simulink model "elevator"  (R2020a)
settings: Solver=FixedStepAuto  StartTime=0.0  StopTime=100  FixedStep=0.001  RelTol=1e-3
settings Model: EnablePacing=on  Creator=Main  LastModifiedBy=Main
settings SolverCC: ZeroCrossAlgorithm=Adaptive
settings DebuggingCC: IgnoredZcDiagnostic=none
settings RTWCC: GenCodeOnly=on  PackageGeneratedCodeAndArtifacts=on
settings GRTTargetCC: MatFileLogging=off
settings ConfigComp: DVTestSuiteOptimization=Auto  DVDetectOutOfBounds=on

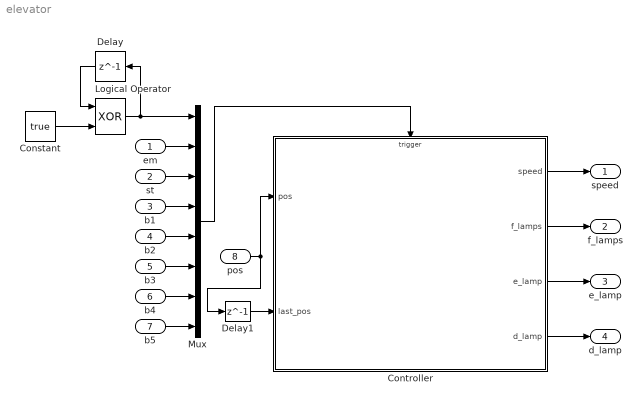
== system elevator ==
  em : Inport
  st : Inport  Port=2
  b1 : Inport  Port=3
  b2 : Inport  Port=4
  b3 : Inport  Port=5
  b4 : Inport  Port=6
  b5 : Inport  Port=7
  pos : Inport  Port=8
  Constant : Constant  Value=true  OutDataTypeStr=boolean
  Controller : Stateflow chart  TreatAsAtomicUnit=on
  Delay : Delay  DelayLength=1
  Delay1 : Delay  DelayLength=1  InitialCondition=1
  Logical Operator : Logic  Operator=XOR  AllPortsSameDT=off  OutDataTypeStr=boolean
  Mux : Mux  Inputs=8
  speed : Outport
  f_lamps : Outport  Port=2
  e_lamp : Outport  Port=3
  d_lamp : Outport  Port=4
  wires:
  Controller/1(speed) -> speed/1
  Controller/3(e_lamp) -> e_lamp/1
  Controller/4(d_lamp) -> d_lamp/1
  Controller/2(f_lamps) -> f_lamps/1
  Logical Operator/1 -> Mux/1, Delay/1
  Mux/1 -> Controller/Trigger
  Constant/1 -> Logical Operator/2
  Delay/1 -> Logical Operator/1
  em/1 -> Mux/2
  b5/1 -> Mux/8
  b4/1 -> Mux/7
  b3/1 -> Mux/6
  b2/1 -> Mux/5
  b1/1 -> Mux/4
  st/1 -> Mux/3
  pos/1 -> Delay1/1, Controller/1(pos)
  Delay1/1 -> Controller/2(last_pos)

== stateflow chart elevator/Controller ==
  settings: sampleTime=0.01  executeAtInitialization=1
  state ControlModule
    state FloorButton [parallel]
      settings: executionOrder=2
      state Buttons
      Buttons -> Buttons [order 1] : B1 /{lamp_state(1); Button}
      (default) -> Buttons
      Buttons -> Buttons [order 5] : B5 /{lamp_state(5);
          |        Button}
      Buttons -> Buttons [order 2] : B2 /{lamp_state(2);
          |         Button}
      Buttons -> Buttons [order 3] : B3 /{lamp_state(3); Button}
      Buttons -> Buttons [order 4] : B4 /{lamp_state(4);
          |         Button}
    state Controller [parallel]
      settings: executionOrder=1
      state Normal
        state Moving
          state FullSpeed
          state Break
            du: speed = target - pos;
          (default) -> FullSpeed
          FullSpeed -> Break [order 1] : [ab(pos - target) < 0.4]
        state Idle
          en: speed = 0;
        state Plan
          en:
          plan();
          speed = direction * MAX_SPEED;
        state Doors
          en:
          f_lamps[target-1] = LAMP_HERE;
          d_lamp = 1;
        state DoorWait
        Idle -> Plan [order 3] : [sumlamps() > 0]
        (default) -> Idle
        Plan -> Moving [order 2] : [at_floor() != target]
        Idle -> Plan [order 1] : Button
        FullSpeed -> Plan [order 2] : Button
        Plan -> Idle [order 1] : [target < 1]
        Idle -> Doors [order 2] : [d_lamp]
        Doors -> Plan : [after(5, sec)]
            | /{d_lamp = 0;
            |   f_lamps[target-1] = LAMP_OFF;}
        Plan -> Doors [order 3] : [at_floor() == target && speed == 0]
        Moving -> DoorWait : [at_floor() == target]
            | /{speed = 0;}
        DoorWait -> Doors : [after(0.5,sec)]
      state Emergency
        en:
        e_lamp = 1;
        speed = 0;
        state WaitForRelease
        state Stabilize
        Stabilize -> WaitForRelease [order 2] : [after(5, sec)]
        Stabilize -> Stabilize [order 1] : [ab(pos - last_pos) > POS_FAULT]
        WaitForRelease -> Stabilize [order 1] : [ab(pos - last_pos) > POS_FAULT]
      (default) -> Normal
      WaitForRelease -> Doors [order 2] : Emergency[d_lamp == 1]
          | /{e_lamp = 0;}
      WaitForRelease -> Normal [order 3] : Emergency[d_lamp == 0]
          | /{e_lamp = 0;}
      Normal -> WaitForRelease [order 1] : Emergency
      Normal -> Stabilize [order 2] : [ab(pos - last_pos) > POS_FAULT]
  (default) -> ControlModule
  data: y function_output double; k function_input double; s function_output int8; v function_output double; x function_input double; speed output double; pos input double; f_lamps output int8 size=5; e_lamp output boolean; LAMP_OFF constant int8 =0; LAMP_ON constant int8 =1; LAMP_TARGET constant int8 =2; LAMP_HERE constant int8 =3; MAX_SPEED constant double =1; target local int8 =-1; direction local double =0; d_lamp output boolean; FLOORS constant int8 =5; last_pos input double =1; POS_FAULT constant double =0.1
  events: TIC input RISING_EDGE_EVENT; Emergency input RISING_EDGE_EVENT; Start input RISING_EDGE_EVENT; B1 input RISING_EDGE_EVENT; B2 input RISING_EDGE_EVENT; B3 input RISING_EDGE_EVENT; B4 input RISING_EDGE_EVENT; Button local RISING_EDGE_EVENT; B5 input RISING_EDGE_EVENT
  function y = at_floor:
    | % calculate which floor the elevator is on
    | % if elevator not at a floor, return -1
    | function y = at_floor()
    |     %y = -1;
    |     %for k = 1:FLOORS
    |     %    if abs(pos - k) < 0.01
    |     %        y = k;
    |     %        return;
    |     %    end
    |     nearest = round(pos);
    |     if abs(pos - nearest) < 0.02
    |         y = nearest;
    |     else
    |         y = -1;
    |     end
    | end
  function plan:
    | % set target of elevator, and update the floor state
    | % since the lamps colour is based on floor state, why not use that?
    | function plan()
    |     old_target = target;    % used to set state of old target from Target to On
    |     % if currently going up, prioritise the up direction
    |     if direction > 0
    |         if look_up(old_target)
    |             % nothing up, look down
    |             if look_down(old_target)
    |                 % nothing down either, elevator is idle
    |                 direction = 0;
    |                 target = int8(-1);
    |             end
    |         end
    |     else
    |         % if going down, or if idle, look down first then up
    |         if look_down(old_target)
    |             if look_up(old_target)
    |                 % noting, elevator is idle
    |                 direction = 0;
    |                 target = int8(-1);
    |             end
    |         end
    |     end
    | end
    | 
    | % look floors above
    | % if no target, returns 1 - otherwise returns 0
    | function no = look_up(old_target)
    |     % just in case elevator is slightly above top floor
    |     % shouldn't happen, but just in case
    |     next_floor = min(ceil(pos+0.5), FLOORS);
    |     no = 1;
    |     % look at above floors, starting with nearest
    |     for k = next_floor:FLOORS
    |         % if floor light is on, or if floor is already target
    |         if f_lamps(k) == LAMP_ON || f_lamps(k) == LAMP_TARGET
    |             % if not target, old target should not be target
    |             % but should still be on
    |             if old_target > 0
    |                 if f_lamps(old_target) == LAMP_TARGET
    |                     f_lamps(old_target) = LAMP_ON;
    |                 end
    |             end
    |             % set as target
    |             f_lamps(k) = LAMP_TARGET;
    |             target = int8(k);
    |             if target ~= at_floor()
    |                 direction = 1;
    |             end
    |             no = 0;
    |             return;
    |         end
    |     end
    | end
    | 
    | % look floors below
    | % if no target, returns 1 - otherwise returns 0
    | function no = look_down(old_target)
    |     % just in case elevator is slightly below bottom floor
    |     % shouldn't happen, but just in case
    |     next_floor = max(floor(pos-0.5), 1);
    |     no = 1;
    |     % look at below floors, starting with nearest
    |     for k = 1:next_floor
    |         ind = int8(next_floor + 1 - k);
    |         % if floor light is on, or if floor is already target
    |         if f_lamps(ind) == LAMP_ON || f_lamps(ind) == LAMP_TARGET
    |             % if not target, old target should not be target
    |             % but should still be on
    |             if old_target > 0
    |                 if f_lamps(old_target) == LAMP_TARGET
    |                     f_lamps(old_target) = LAMP_ON;
    |                 end
    |             end
    |             % set as target
    |             f_lamps(ind) = LAMP_TARGET;
    |             target = ind;
    |             if target ~= at_floor()
    |                 direction = -1;
    |             end
    |             no = 0;
    |             return;
    |         end
    |     end
    | end
  function lamp_state(k):
    | % toggle state of lamp k between on and off
    | % ignored if lamp is in state target or here
    | function lamp_state(k)
    |     %for k=1:FLOORS
    |         if f_lamps(k) == LAMP_OFF
    |             f_lamps(k) = LAMP_ON;
    |         end
    |     %end
    | end
  function s = sumlamps:
    | function s = sumlamps()
    |     s = f_lamps(1) + f_lamps(2) + f_lamps(3) + f_lamps(4) + f_lamps(5);
    | end
  function v = ab(x):
    | function v = ab(x)
    |     v = abs(x);
    | end
